simulink model "trackCircle2"  (R2020a)
settings: Solver=VariableStepAuto  StartTime=0.0  StopTime=P  RelTol=1e-8
undefined symbols (not defined in the file or in its folder): den_latRot, num_latRot, sensor_gain, V_avg
libraries: simulink x2
settings Model: Creator=Tomo  LastModifiedBy=Tomo

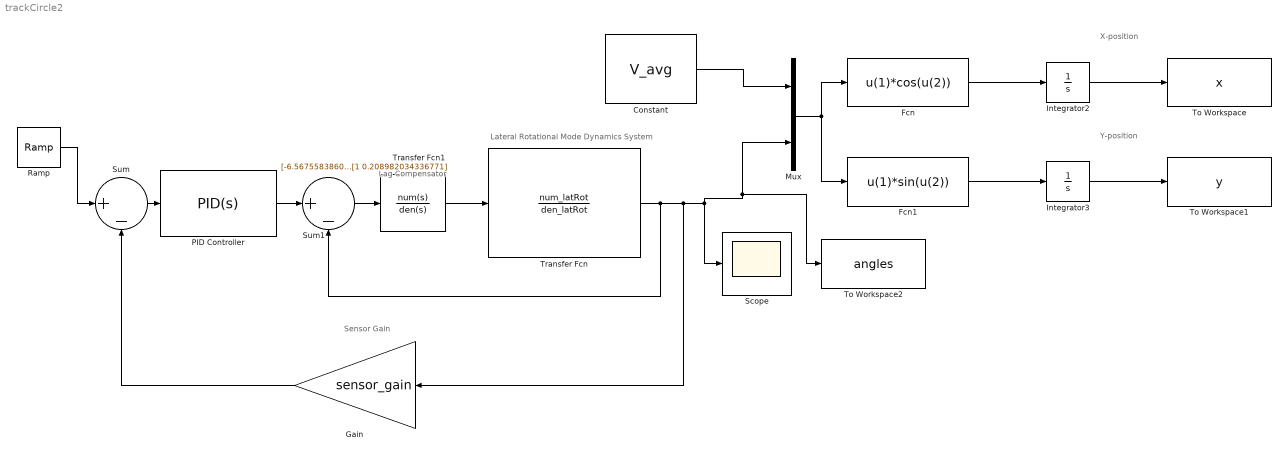
== system trackCircle2 ==
  note: Y-position
  note: X-position
  note: Lateral Rotational Mode Dynamics System
  note: Sensor Gain
  note: Lag Compensator
  Constant : Constant  Value=V_avg
  Fcn : Fcn  Expr=u(1)*cos(u(2))
  Fcn1 : Fcn  Expr=u(1)*sin(u(2))
  Gain : Gain  Gain=sensor_gain
  Integrator2 : Integrator
  Integrator3 : Integrator
  Mux : Mux  Inputs=2
  PID Controller : simulink/Continuous/PID Controller  Controller=PID  Form=Parallel  TimeDomain=Continuous-time  UseExternalTs=off  SampleTime=-1  IntegratorMethod=Forward Euler  FilterMethod=Forward Euler  ControllerParametersSource=internal  P=-0.500255559170676  I=1.6854356948078  D=6.59101770729751  UseFilter=on  N=3.36713693817372  TunerSelectOption=Transfer Function Based (PID Tuner App)  InitialConditionSource=internal  InitialConditionForIntegrator=0  InitialConditionForFilter=0  DifferentiatorICPrevScaledInput=0  ExternalReset=none  TrackingMode=off  Kt=1  LimitOutput=off  UpperSaturationLimit=inf  LowerSaturationLimit=-inf  LinearizeAsGain=on  AntiWindupMode=none  Kb=1  POutMin=[]  POutMax=[]  IOutMin=[]  IOutMax=[]  DOutMin=[]  DOutMax=[]  NOutMin=[]  NOutMax=[]  SumOutMin=[]  SumOutMax=[]  SaturationOutMin=[]  SaturationOutMax=[]  PParamMin=[]  PParamMax=[]  IParamMin=[]  IParamMax=[]  DParamMin=[]  DParamMax=[]  NParamMin=[]  NParamMax=[]  KbParamMin=[]  KbParamMax=[]  KtParamMin=[]  KtParamMax=[]  KbOutMin=[]  KbOutMax=[]  KtOutMin=[]  KtOutMax=[]  IntegratorOutMin=[]  IntegratorOutMax=[]  FilterOutMin=[]  FilterOutMax=[]  SumI1OutMin=[]  SumI1OutMax=[]  SumI2OutMin=[]  SumI2OutMax=[]  SumI3OutMin=[]  SumI3OutMax=[]  SumI4OutMin=[]  SumI4OutMax=[]  SumDOutMin=[]  SumDOutMax=[]  DifferentiatorOutMin=[]  DifferentiatorOutMax=[]  FilterDiffOutCoefMin=[]  FilterDiffOutCoefMax=[]  ReciprocalOutMin=[]  ReciprocalOutMax=[]  SumDenOutMin=[]  SumDenOutMax=[]  SumNumOutMin=[]  SumNumOutMax=[]  DivideOutMin=[]  DivideOutMax=[]  UdiffTsProdOutMin=[]  UdiffTsProdOutMax=[]  NTsProdOutMin=[]  NTsProdOutMax=[]  UintegralTsProdOutMin=[]  UintegralTsProdOutMax=[]  UngainTsProdOutMin=[]  UngainTsProdOutMax=[]  IntegratorContinuousStateAttributes=''  IntegratorStateMustResolveToSignalObject=off  IntegratorRTWStateStorageClass=Auto  FilterContinuousStateAttributes=''  FilterStateMustResolveToSignalObject=off  FilterRTWStateStorageClass=Auto  ParallelPVariant=InternalParameters  IdealPVariant=Disabled  IVariant=InternalParameters  DVariant=InternalParameters  IntegratorVariant=Continuous  SatVariant=Disabled  AWVariant=Passthrough  PCopyVariant=Disabled  TRVariant=Disabled  FdbkBlocksVariant=Forward  IdealPFdbkVariant=Disabled  SatFdbkVariant=Disabled  DerivativeFilterVariant=ContFilter  NVariant=InternalParameters  NCopyVariant=Disabled  FilterICVariant=InternalICsFilter  IntegratorICVariant=InternalICs  ExternalResetVariant=Disabled  TRSumVariant=Passthrough  SumFdbkVariant=Disabled  SumVariant=Sum_PID  TsampFilterVariant=InternalTs  TsampNgainVariant=Passthrough  TsampIntegralVariant=Passthrough
  Ramp : simulink/Sources/Ramp  slope=0.3/8  start=0  InitialOutput=0
  Scope : Scope
  Sum : Sum  Inputs=|+-
  Sum1 : Sum  Inputs=|+-
  To Workspace : ToWorkspace  VariableName=x  SaveFormat=Structure With Time  SampleTime=-1
  To Workspace1 : ToWorkspace  VariableName=y  SaveFormat=Structure With Time  SampleTime=-1
  To Workspace2 : ToWorkspace  VariableName=angles  SaveFormat=Structure With Time  SampleTime=-1
  Transfer Fcn : TransferFcn  Numerator=num_latRot  Denominator=den_latRot
  Transfer Fcn1 : TransferFcn  Numerator=[-6.56755838601913e-09 31.2970399061581]  Denominator=[1 0.208982034336771]
  wires:
  Constant/1 -> Mux/1
  Mux/1 -> Fcn/1, Fcn1/1
  Integrator3/1 -> To Workspace1/1
  Fcn/1 -> Integrator2/1
  Integrator2/1 -> To Workspace/1
  Fcn1/1 -> Integrator3/1
  Gain/1 -> Sum/2
  Transfer Fcn1/1 -> Transfer Fcn/1
  Sum1/1 -> Transfer Fcn1/1
  Sum/1 -> PID Controller/1
  PID Controller/1 -> Sum1/1
  Transfer Fcn/1 -> Sum1/2, Gain/1, To Workspace2/1, Mux/2, Scope/1
  Ramp/1 -> Sum/1
